simulink model "integrating_model"  (R2020a)
settings: Solver=FixedStepAuto  StartTime=0.0  StopTime=tn(end)  FixedStep=0.001  RelTol=1e-3
values from neighbouring files (symbols this model uses):
  a1 = 1    [Link_Model_3.m]    (also in Manipulator.m = 3)
  a2 = 1    [Link_Model_3.m]    (also in Manipulator.m = 3)
  DMP_Par = readtable(fName)    [load_weights.m]
  k1 = 300    [Manipulator.m]
  k2 = 40    [Manipulator.m]
  q = v+2*pi    [Link_Model_3.m]    (also in Manipulator.m = [theta1,theta2])
  q0 = two_link_Inv_Kin(q(1,1),q(1,2),a1,a2,1)    [Manipulator.m]
libraries: simulink x2
settings Model: Creator=sirius  LastModifiedBy=sirius

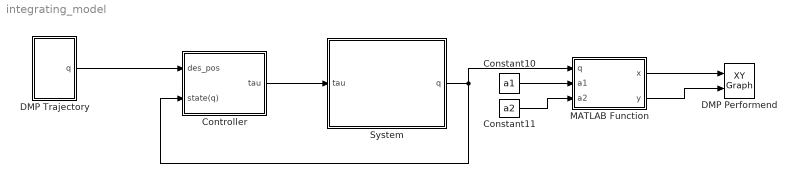
== system integrating_model ==
  Constant10 : Constant  Value=a1
  Constant11 : Constant  Value=a2
  Controller : Subsystem
  DMP Performend : simulink/Sinks/XY Graph  xmin=-3  xmax=3  ymin=-3  ymax=3  st=-1
  DMP Trajectory : Subsystem
  MATLAB Function : MATLAB Function  TreatAsAtomicUnit=on
  System : Subsystem
  wires:
  DMP Trajectory/1(q) -> Controller/1(des_pos)
  Controller/1(tau) -> System/1(tau)
  System/1(q) -> Controller/2(state(q)), MATLAB Function/1(q)
  Constant10/1 -> MATLAB Function/2(a1)
  Constant11/1 -> MATLAB Function/3(a2)
  MATLAB Function/1(x) -> DMP Performend/1
  MATLAB Function/2(y) -> DMP Performend/2

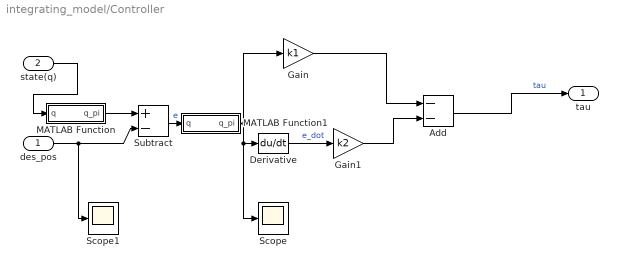
== system integrating_model/Controller ==
  des_pos : Inport
  state(q) : Inport  Port=2
  Add : Sum  Inputs=--
  Derivative : Derivative
  Gain : Gain  Gain=k1
  Gain1 : Gain  Gain=k2
  MATLAB Function : MATLAB Function  TreatAsAtomicUnit=on
  MATLAB Function1 : MATLAB Function  TreatAsAtomicUnit=on
  Scope : Scope
  Scope1 : Scope
  Subtract : Sum  Inputs=+-
  tau : Outport
  wires:
  Gain/1 -> Add/1
  Gain1/1 -> Add/2
  Add/1 -> tau/1  "tau"
  des_pos/1 -> Subtract/2, Scope1/1
  Derivative/1 -> Gain1/1  "e_dot"
  state(q)/1 -> MATLAB Function/1(q)
  MATLAB Function/1(q_pi) -> Subtract/1
  Subtract/1 -> MATLAB Function1/1(q)  "e"
  MATLAB Function1/1(q_pi) -> Scope/1, Derivative/1, Gain/1

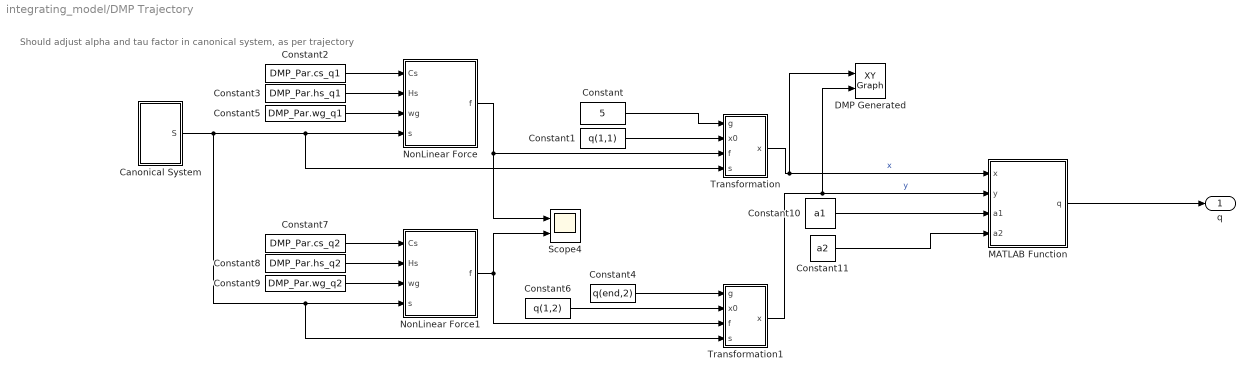
== system integrating_model/DMP Trajectory ==
  note: Should adjust alpha and tau factor in canonical system, as per trajectory
  Canonical System : Subsystem
  Constant : Constant  Value=5
  Constant1 : Constant  Value=q(1,1)
  Constant10 : Constant  Value=a1
  Constant11 : Constant  Value=a2
  Constant2 : Constant  Value=DMP_Par.cs_q1  VectorParams1D=off
  Constant3 : Constant  Value=DMP_Par.hs_q1  VectorParams1D=off
  Constant4 : Constant  Value=q(end,2)
  Constant5 : Constant  Value=DMP_Par.wg_q1  VectorParams1D=off
  Constant6 : Constant  Value=q(1,2)
  Constant7 : Constant  Value=DMP_Par.cs_q2  VectorParams1D=off
  Constant8 : Constant  Value=DMP_Par.hs_q2  VectorParams1D=off
  Constant9 : Constant  Value=DMP_Par.wg_q2  VectorParams1D=off
  DMP Generated : simulink/Sinks/XY Graph  xmin=-3  xmax=3  ymin=-3  ymax=3  st=-1
  MATLAB Function : MATLAB Function  TreatAsAtomicUnit=on
  NonLinear Force : MATLAB Function  TreatAsAtomicUnit=on
  NonLinear Force1 : MATLAB Function  TreatAsAtomicUnit=on
  Scope4 : Scope  NumInputPorts=2
  Transformation : Subsystem
  Transformation1 : Subsystem
  q : Outport
  wires:
  Constant/1 -> Transformation/1(g)
  NonLinear Force1/1(f) -> Transformation1/3(f), Scope4/2
  Constant3/1 -> NonLinear Force/2(Hs)
  Constant1/1 -> Transformation/2(x0)
  Canonical System/1(S) -> Transformation1/4(s), NonLinear Force1/4(s), Transformation/4(s), NonLinear Force/4(s)
  Transformation/1(x) -> DMP Generated/1, MATLAB Function/1(x)  "x"
  Constant9/1 -> NonLinear Force1/3(wg)
  Constant6/1 -> Transformation1/2(x0)
  NonLinear Force/1(f) -> Scope4/1, Transformation/3(f)
  Constant7/1 -> NonLinear Force1/1(Cs)
  Constant2/1 -> NonLinear Force/1(Cs)
  Constant5/1 -> NonLinear Force/3(wg)
  Constant8/1 -> NonLinear Force1/2(Hs)
  Constant4/1 -> Transformation1/1(g)
  Transformation1/1(x) -> DMP Generated/2, MATLAB Function/2(y)  "y"
  Constant10/1 -> MATLAB Function/3(a1)
  Constant11/1 -> MATLAB Function/4(a2)
  MATLAB Function/1(q) -> q/1

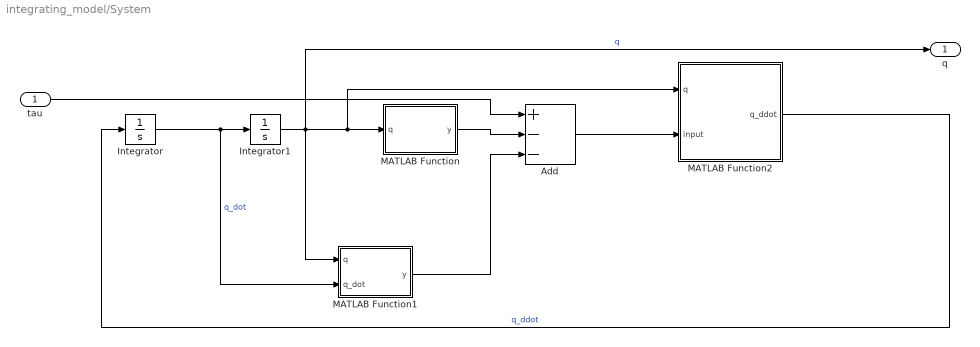
== system integrating_model/System ==
  tau : Inport
  Add : Sum  Inputs=+--
  Integrator : Integrator  InitialCondition=q0
  Integrator1 : Integrator  InitialCondition=q0
  MATLAB Function : MATLAB Function  TreatAsAtomicUnit=on
  MATLAB Function1 : MATLAB Function  TreatAsAtomicUnit=on
  MATLAB Function2 : MATLAB Function  TreatAsAtomicUnit=on
  q : Outport
  wires:
  MATLAB Function1/1(y) -> Add/3
  Integrator1/1 -> MATLAB Function1/1(q), q/1, MATLAB Function2/1(q), MATLAB Function/1(q)  "q"
  tau/1 -> Add/1
  Integrator/1 -> MATLAB Function1/2(q_dot), Integrator1/1  "q_dot"
  MATLAB Function2/1(q_ddot) -> Integrator/1  "q_ddot"
  Add/1 -> MATLAB Function2/2(input)
  MATLAB Function/1(y) -> Add/2

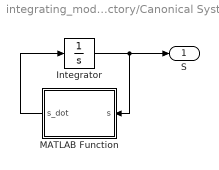
== system integrating_model/DMP Trajectory/Canonical System ==
  Integrator : Integrator  InitialCondition=1
  MATLAB Function : MATLAB Function  TreatAsAtomicUnit=on
  S : Outport
  wires:
  MATLAB Function/1(s_dot) -> Integrator/1
  Integrator/1 -> MATLAB Function/1(s), S/1

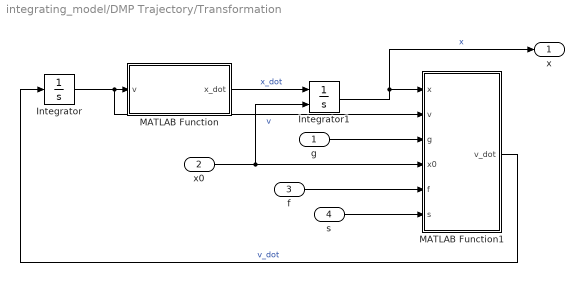
== system integrating_model/DMP Trajectory/Transformation ==
  g : Inport
  x0 : Inport  Port=2
  f : Inport  Port=3
  s : Inport  Port=4
  Integrator : Integrator
  Integrator1 : Integrator  InitialConditionSource=external  InitialCondition=q(1,1)
  MATLAB Function : MATLAB Function  TreatAsAtomicUnit=on
  MATLAB Function1 : MATLAB Function  TreatAsAtomicUnit=on
  x : Outport
  wires:
  Integrator1/1 -> x/1, MATLAB Function1/1(x)  "x"
  f/1 -> MATLAB Function1/5(f)
  x0/1 -> Integrator1/2, MATLAB Function1/4(x0)
  MATLAB Function1/1(v_dot) -> Integrator/1  "v_dot"
  Integrator/1 -> MATLAB Function1/2(v), MATLAB Function/1(v)  "v"
  g/1 -> MATLAB Function1/3(g)
  MATLAB Function/1(x_dot) -> Integrator1/1  "x_dot"
  s/1 -> MATLAB Function1/6(s)

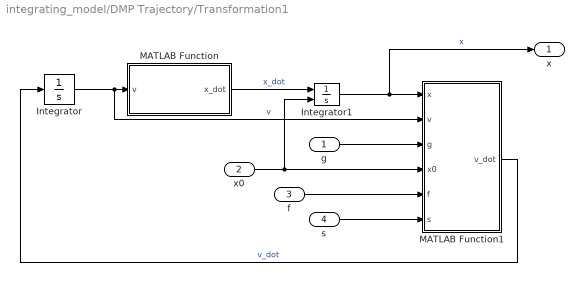
== system integrating_model/DMP Trajectory/Transformation1 ==
  g : Inport
  x0 : Inport  Port=2
  f : Inport  Port=3
  s : Inport  Port=4
  Integrator : Integrator
  Integrator1 : Integrator  InitialConditionSource=external  InitialCondition=q(1,1)
  MATLAB Function : MATLAB Function  TreatAsAtomicUnit=on
  MATLAB Function1 : MATLAB Function  TreatAsAtomicUnit=on
  x : Outport
  wires:
  Integrator1/1 -> x/1, MATLAB Function1/1(x)  "x"
  f/1 -> MATLAB Function1/5(f)
  x0/1 -> Integrator1/2, MATLAB Function1/4(x0)
  MATLAB Function1/1(v_dot) -> Integrator/1  "v_dot"
  Integrator/1 -> MATLAB Function1/2(v), MATLAB Function/1(v)  "v"
  g/1 -> MATLAB Function1/3(g)
  MATLAB Function/1(x_dot) -> Integrator1/1  "x_dot"
  s/1 -> MATLAB Function1/6(s)

== matlab function integrating_model/System/MATLAB Function2 ==
  data: q input; input input; q_ddot output
function q_ddot = M_inverse(q,input)
% M = [3 + 2*cos(q(2)), 1 + cos(q(2));
%     1 + cos(q(2)), 1;];
M =  [ (9*cos(q(2)))/2 + 27/4, (9*cos(q(2)))/4 + 9/4;
  (9*cos(q(2)))/4 + 9/4,                 9/4];

q_ddot = inv(M)*input;
% q_ddot = M/input;

== matlab function integrating_model/MATLAB Function ==
  data: x output; q input; y output; a1 input; a2 input
function [x,y] = fcn(q,a1,a2)
x = a1*cos(q(1)) + a2*cos(q(1)+q(2));
y = a1*sin(q(1)) + a2*sin(q(1) + q(2));
end

== matlab function integrating_model/DMP Trajectory/Transformation/MATLAB Function ==
  data: v input; x_dot output
function x_dot = Eq2(v)
tau = 1;
x_dot = v/tau;

== matlab function integrating_model/Controller/MATLAB Function ==
  data: q input; q_pi output
function q_pi = fcn(q)
q_pi = [atan2(sin(q(1)),cos(q(1)));
        atan2(sin(q(2)),cos(q(2)));];
end

== matlab function integrating_model/Controller/MATLAB Function1 ==
  data: q input; q_pi output
function q_pi = fcn(q)
q_pi = [atan2(sin(q(1)),cos(q(1)));
        atan2(sin(q(2)),cos(q(2)));];
end

== matlab function integrating_model/DMP Trajectory/Canonical System/MATLAB Function ==
  data: s input; s_dot output
function s_dot = fcn(s)
tau  = 1; alp_s = 0.1;
s_dot = -alp_s/tau*s;

== matlab function integrating_model/DMP Trajectory/Transformation/MATLAB Function1 ==
  data: x input; v_dot output; v input; g input; x0 input; f input; s input
function v_dot = Eq1(x,v,g,x0,f,s)
K = 1;
D = sqrt(4*K);
tau = 1;
v_dot =  (K*(g - x) - D*v -K*(g - x0)*s +K*f)/tau;
end

== matlab function integrating_model/DMP Trajectory/NonLinear Force ==
  data: Cs input; f output; Hs input; wg input; s input
function f = force(Cs,Hs,wg,s)
    sVal = 0;sWVal = 0;
    for i = 1:length(Cs(:,1))
        sVal = sVal + exp(-Hs(i,1)*((s - Cs(i,1))^2));
        sWVal = sWVal + wg(i,1)*exp(-Hs(i,1)*((s - Cs(i,1))^2));
    end
%     sVal = exp(-Hs(1,1)*((s - Cs(1,1))^2)) + exp(-Hs(1,2)*((s - Cs(1,2))^2)) +  exp(-Hs(1,3)*((s - Cs(1,3))^2)) + exp(-Hs(1,4)*((s - Cs(1,4))^2)) + exp(-Hs(1,5)*((s - Cs(1,5))^2)) +exp(-Hs(1,6)*((s - Cs(1,6))^2)) + exp(-Hs(1,7)*((s - Cs(1,7))^2)) + exp(-Hs(1,8)*((s - Cs(1,8))^2)) + exp(-Hs(1,9)*((s - Cs(1,9))^2)) + exp(-Hs(1,10)*((s - Cs(1,10))^2)) + exp(-Hs(1,11)*((s - Cs(1,11))^2)) + exp(-Hs(1,12)*((s - Cs(1,12))^2)) + exp(-Hs(1,13)*((s - Cs(1,13))^2)) + exp(-Hs(1,14)*((s - Cs(1,14))^2)) + exp(-Hs(1,15)*((s - Cs(1,15))^2)) + exp(-Hs(1,16)*((s - Cs(1,16))^2)) + exp(-Hs(1,17)*((s - Cs(1,17))^2)) + exp(-Hs(1,18)*((s - Cs(1,18))^2)) + exp(-Hs(1,19)*((s - Cs(1,19))^2)) + exp(-Hs(1,20)*((s - Cs(1,20))^2)) ;
%     sWVal = wg(1,1)*exp(-Hs(1,1)*((s - Cs(1,1))^2)) + wg(2,1)*exp(-Hs(1,2)*((s - Cs(1,2))^2)) +  wg(3,1)*exp(-Hs(1,3)*((s - Cs(1,3))^2)) + wg(4,1)*exp(-Hs(1,4)*((s - Cs(1,4))^2)) + wg(5,1)*exp(-Hs(1,5)*((s - Cs(1,5))^2)) + wg(6,1)*exp(-Hs(1,6)*((s - Cs(1,6))^2)) + wg(7,1)*exp(-Hs(1,7)*((s - Cs(1,7))^2)) + wg(8,1)*exp(-Hs(1,8)*((s - Cs(1,8))^2)) + wg(9,1)*exp(-Hs(1,9)*((s - Cs(1,9))^2)) + wg(10,1)*exp(-Hs(1,10)*((s - Cs(1,10))^2)) + wg(11,1)*exp(-Hs(1,11)*((s - Cs(1,11))^2)) + wg(12,1)*exp(-Hs(1,12)*((s - Cs(1,12))^2)) + wg(13,1)*exp(-Hs(1,13)*((s - Cs(1,13))^2)) + wg(14,1)*exp(-Hs(1,14)*((s - Cs(1,14))^2)) + wg(15,1)*exp(-Hs(1,15)*((s - Cs(1,15))^2)) + wg(16,1)*exp(-Hs(1,16)*((s - Cs(1,16))^2)) + wg(17,1)*exp(-Hs(1,17)*((s - Cs(1,17))^2)) + wg(18,1)*exp(-Hs(1,18)*((s - Cs(1,18))^2)) + wg(19,1)*exp(-Hs(1,19)*((s - Cs(1,19))^2)) + wg(20,1)*exp(-Hs(1,20)*((s - Cs(1,20))^2)) ;
    f = (sWVal*s)/sVal;
end

== matlab function integrating_model/DMP Trajectory/NonLinear Force1 ==
  data: Cs input; f output; Hs input; wg input; s input
function f = force(Cs,Hs,wg,s)
    sVal = 0;sWVal = 0;
    for i = 1:length(Cs(:,1))
        sVal = sVal + exp(-Hs(i,1)*((s - Cs(i,1))^2));
        sWVal = sWVal + wg(i,1)*exp(-Hs(i,1)*((s - Cs(i,1))^2));
    end
%     sVal = exp(-Hs(1,1)*((s - Cs(1,1))^2)) + exp(-Hs(1,2)*((s - Cs(1,2))^2)) +  exp(-Hs(1,3)*((s - Cs(1,3))^2)) + exp(-Hs(1,4)*((s - Cs(1,4))^2)) + exp(-Hs(1,5)*((s - Cs(1,5))^2)) +exp(-Hs(1,6)*((s - Cs(1,6))^2)) + exp(-Hs(1,7)*((s - Cs(1,7))^2)) + exp(-Hs(1,8)*((s - Cs(1,8))^2)) + exp(-Hs(1,9)*((s - Cs(1,9))^2)) + exp(-Hs(1,10)*((s - Cs(1,10))^2)) + exp(-Hs(1,11)*((s - Cs(1,11))^2)) + exp(-Hs(1,12)*((s - Cs(1,12))^2)) + exp(-Hs(1,13)*((s - Cs(1,13))^2)) + exp(-Hs(1,14)*((s - Cs(1,14))^2)) + exp(-Hs(1,15)*((s - Cs(1,15))^2)) + exp(-Hs(1,16)*((s - Cs(1,16))^2)) + exp(-Hs(1,17)*((s - Cs(1,17))^2)) + exp(-Hs(1,18)*((s - Cs(1,18))^2)) + exp(-Hs(1,19)*((s - Cs(1,19))^2)) + exp(-Hs(1,20)*((s - Cs(1,20))^2)) ;
%     sWVal = wg(1,1)*exp(-Hs(1,1)*((s - Cs(1,1))^2)) + wg(2,1)*exp(-Hs(1,2)*((s - Cs(1,2))^2)) +  wg(3,1)*exp(-Hs(1,3)*((s - Cs(1,3))^2)) + wg(4,1)*exp(-Hs(1,4)*((s - Cs(1,4))^2)) + wg(5,1)*exp(-Hs(1,5)*((s - Cs(1,5))^2)) + wg(6,1)*exp(-Hs(1,6)*((s - Cs(1,6))^2)) + wg(7,1)*exp(-Hs(1,7)*((s - Cs(1,7))^2)) + wg(8,1)*exp(-Hs(1,8)*((s - Cs(1,8))^2)) + wg(9,1)*exp(-Hs(1,9)*((s - Cs(1,9))^2)) + wg(10,1)*exp(-Hs(1,10)*((s - Cs(1,10))^2)) + wg(11,1)*exp(-Hs(1,11)*((s - Cs(1,11))^2)) + wg(12,1)*exp(-Hs(1,12)*((s - Cs(1,12))^2)) + wg(13,1)*exp(-Hs(1,13)*((s - Cs(1,13))^2)) + wg(14,1)*exp(-Hs(1,14)*((s - Cs(1,14))^2)) + wg(15,1)*exp(-Hs(1,15)*((s - Cs(1,15))^2)) + wg(16,1)*exp(-Hs(1,16)*((s - Cs(1,16))^2)) + wg(17,1)*exp(-Hs(1,17)*((s - Cs(1,17))^2)) + wg(18,1)*exp(-Hs(1,18)*((s - Cs(1,18))^2)) + wg(19,1)*exp(-Hs(1,19)*((s - Cs(1,19))^2)) + wg(20,1)*exp(-Hs(1,20)*((s - Cs(1,20))^2)) ;
    f = (sWVal*s)/sVal;

end

== matlab function integrating_model/DMP Trajectory/Transformation1/MATLAB Function ==
  data: v input; x_dot output
function x_dot = Eq2(v)
tau = 1;
x_dot = v/tau;

== matlab function integrating_model/DMP Trajectory/Transformation1/MATLAB Function1 ==
  data: x input; v_dot output; v input; g input; x0 input; f input; s input
function v_dot = Eq1(x,v,g,x0,f,s)
K = 1;
D = sqrt(4*K);
tau = 1;
v_dot =  (K*(g - x) - D*v -K*(g - x0)*s +K*f)/tau;

== matlab function integrating_model/DMP Trajectory/MATLAB Function ==
  data: x input; y input; q output; a1 input; a2 input
function q = Inv_Kin(x, y,a1,a2)
    s= 1;
    theta2 = s*acos((x^2 + y^2 - a1^2 - a2^2)/(2*a1*a2));    
    theta1 = atan2(y,x) - atan2(a2*sin(theta2),a1+a2*cos(theta2));
    q = [theta1;
         theta2;];
     
end

== matlab function integrating_model/System/MATLAB Function ==
  data: q input; y output
function y = G(q)
g = 9.81; %ms^-2
% y = [2*g*cos(q(1)) + g*cos(q(1)+q(2));
%      g*cos(q(1)+q(2));
%      ];
y = [0;0];

== matlab function integrating_model/System/MATLAB Function1 ==
  data: q input; y output; q_dot input
function y = V(q,q_dot)
% y  = [-2*q_dot(1)*q_dot(2)*sin(q(2)) - (q_dot(2)^2)*sin(q(2));
%       (q_dot(1)^2)*sin(q(2));
%       ];
y = [-sin(q(2))*((9*q_dot(2)^2)/4 + (9*q_dot(1)*q_dot(2))/2);
                    (9*q_dot(1)^2*sin(q(2)))/4];
end
